simulink model "HM_to_Unity_2013a"  (R2013a)
settings: Solver=FixedStepDiscrete  StartTime=0.0  StopTime=Inf  FixedStep=0.0004  RelTol=1e-3
InitFcn:
  | SampleTime = 0.0004;
  | sampleTime = 0.0004;
undefined symbols (not defined in the file or in its folder): DiscIntNeverNeededParam
libraries: simulink x26, dspsigops x10, xpcmeasurementcomputinglib x7, xpclib x6, dspmtrx3 x4, etargetslib x2, hm_iointerface_lib x2, hm_control_lib x2, sensors_jr3_lib x1
(part 2 of 2)

== matlab function HM_to_Unity_2013a/Subsystem/GotoBlock/compare ==
  data: sig input; f output; comp input; eps input
function f = fcn(sig,comp,eps)
% This block supports the Embedded MATLAB subset.
% See the help menu for details. 

dVec=comp-sig;
delta=norm(dVec);
if (delta<eps)
    f=1;
else
    f=0;
end

== stateflow chart HM_to_Unity_2013a/Robot State Control/Chart2 ==
  state MotorOn1
    en:State=-2;
    en:inPosReset=0;
    count=0;
    du:State=-2;
    du:inPosReset=1;
    ex:inPosReset=0;
  state MotorOn
    en:State=-2;
    count=0;
    du:count=count+1;
    du:State=-2;
  state WaitNewState
    count=0;
    du:count=count+1;
  state DeadMan
    en:State=-1;
    count=0;
    du:State=-1;
  state KeepPos
    en:State=0;
    count=0;
    du:State=0;
    du:count=count+1;
  state FreeSpace
    en:State=1;
    count=0;
    du:State=1;
    du:count=count+1;
  state GoTo1
    en:State=3;
    count=0;
    du:State=3;
    du:count=count+1;
  state Main
    en:State=2;
    count=0;
    du:State=2;
    du:count=count+1;
  state GoTo
    en:State=3;
    count=0;
    du:State=3;
    du:count=count+1;
  (default) -> MotorOn1
  DeadMan -> MotorOn : [DMSwitch==1]
  MotorOn1 -> DeadMan [order 1] : [DMSwitch==0]
  MotorOn -> KeepPos [order 2] : [F0==1 && reset==1]
  MotorOn -> DeadMan [order 1] : [DMSwitch==0]
  MotorOn1 -> KeepPos [order 2] : [F0==1 && reset==1]
  WaitNewState -> KeepPos [order 1] : [F0==1 && reset==1]
  KeepPos -> DeadMan [order 1] : [DMSwitch==0]
  GoTo -> KeepPos [order 1] : [F0==1 && reset==1]
  KeepPos -> WaitNewState [order 2] : [count>2000]
  Main -> KeepPos [order 1] : [F0==1 && reset==1]
  WaitNewState -> FreeSpace [order 2] : [F1==1 && reset==1]
  FreeSpace -> DeadMan [order 1] : [DMSwitch==0]
  FreeSpace -> WaitNewState [order 2] : [count>2000]
  GoTo1 -> DeadMan [order 1] : [DMSwitch==0]
  WaitNewState -> GoTo1 [order 3] : [F2==1 && reset==1]
  GoTo1 -> Main [order 2] : [finishedTask==1]
  GoTo1 -> Main [order 3] : [F2==1 && reset==1 && (count>13000) ]
  Main -> DeadMan [order 2] : [DMSwitch==0]
  WaitNewState -> GoTo [order 4] : [F3==1 && reset==1]
  GoTo -> DeadMan [order 2] : [DMSwitch==0]
  WaitNewState -> DeadMan [order 5] : [DMSwitch==0]
  data: State output double; count local uint32; finishedTask input boolean; F0 input double; F1 input double; F2 input double; F3 input double; reset input double; DMSwitch input double; inPosReset output double =0

== stateflow chart HM_to_Unity_2013a/Robot State Control/Chart1 ==
  state Up
    en:handleType=0
  state Down
    en:handleType=1
  (default) -> Up
  Up -> Down : [Switch==1 && after(1,sec)]
  Down -> Up : [Switch==1 && after(1,sec)]
  data: Switch input; handleType output double

== matlab function HM_to_Unity_2013a/HapticMaster inputs/Balanca enkoderji/Sile na rockah ==
  data: Fd input; Fdo output
function Fdo    = fcn(Fd)
%#codegen

Fdo = Fd;

Fdo(1) = Fd(3);
Fdo(2) = Fd(1);
Fdo(3) = -Fd(2);

% Flo(1) = Fl(2);
% Flo(2) = -Fl(3);
% Flo(3) = Fl(1);
% 
% Fdo(1) = -Fd(2);
% Fdo(2) = Fd(3);
% Fdo(3) = Fd(1);

== matlab function HM_to_Unity_2013a/HapticMaster inputs/Sila_na_vhu/Sila na vrhu ==
  data: rot_mali input; rot_velik input; F output; Fd input
function F   = fcn(rot_mali, rot_velik, Fd)
%#codegen

Rm=[1 0 0;0 cos(rot_velik) -sin(rot_velik);0 sin(rot_velik) cos(rot_velik)];
F=Rm*Fd;

== matlab function HM_to_Unity_2013a/Main ==
  data: Unity_World_Pos output; Unity_Scale output; UnityAngles output; inputWorldPos input; inputMotors input; getJointPos input; TargetNumber input; TargetPos output; Color output; OutputTarget output; State output; ListOfTargets input; ListOfTargetsForSecondExp input; ListOfTarget3rdExp input; NumOfTarRep input; angleofJoint output
function [Unity_World_Pos,Unity_Scale,UnityAngles,TargetPos,Color,OutputTarget,State,angleofJoint]= Main(inputWorldPos,inputMotors,getJointPos,TargetNumber,ListOfTargets,ListOfTargetsForSecondExp,ListOfTarget3rdExp,NumOfTarRep)
% This block supports the Embedded MATLAB subset.
% See the help menu for details. 
 State = -1;

Color=0;

%Converting axis
aim_x = inputWorldPos(2);
aim_y = inputWorldPos(3);
scaleofAim = inputWorldPos(1);

%Deviation of angles from handle
anglefor2nd = inputMotors(1);
angleofAim = inputMotors(2);

joint_y = getJointPos(2);
joint_x = getJointPos(1);
if (joint_y < 0)
    joint_y=joint_y;
end


%angleofJoint =atan (joint_y/joint_x)*180/pi;

angleofJoint = joint_y*180/pi;


Unity_X= aim_x ;
Unity_Y = aim_y ;
%Unity_Scale  = (scaleofAim*100)+23;
Unity_Scale= scaleofAim;
angleofAim = angleofAim* 180/pi;
anglefor2nd = anglefor2nd *180/pi;



Unity_World_Pos =[Unity_X,Unity_Y];



%Third row means angle of object and 4th one means scale of object
%%ListOfTargets=[FirstT_x,FirstT_y,30,1;SecondT_x,SecondT_y,0,1.5;ThirdT_x,ThirdT_y,0,1;FourT_x,FourT_y,0,1];
%ListOfTargets=[4.1,-3.7;5.5,-4];
%ExpType=ExpT;

% ka =1;
% if (ka ==1)
% NumberOfTarget = NumOfTarRep (1);
% NumberOfRepeatation = NumOfTarRep (2);
% %size=NumberOfTarget*5;
% OutputTarget = zeros (NumberOfTarget,NumberOfRepeatation);
% else
%     OutputTarget = zeros (1,1);
% end

Deviation = NumOfTarRep(4);
DeviationForScale = NumOfTarRep(5);
DevForAngle=NumOfTarRep(6);
DevForAngle2=NumOfTarRep(7);

ExpType =NumOfTarRep (3);

if (ExpType==1)
    
    UnityAngles = [angleofAim,anglefor2nd];
    OutputTarget = ListOfTargets;
    TargetPos = ListOfTargets (TargetNumber,:);
    if ((Unity_X >TargetPos(1)-Deviation) && ( Unity_Y>TargetPos(2)-Deviation) && (Unity_X<TargetPos(1)+Deviation) && (Unity_Y<TargetPos(2)+Deviation) && (Unity_Scale<TargetPos(4)+DeviationForScale) && (Unity_Scale > TargetPos(4)-DeviationForScale)&&(angleofAim <TargetPos(3)+DevForAngle)&&(angleofAim >TargetPos(3)-DevForAngle))
    %|| (colorCounter>=1 && 100>colorCounter)

State = 1;
Color=1;
%colorCounter = colorCounter+1;
%else
 %   colorCounter =0;
    
elseif (Unity_Scale<TargetPos(4)+DeviationForScale) && (Unity_Scale > TargetPos(4)-DeviationForScale)
    
    Color=2;
   end
elseif (ExpType==3)
    
    limit = anglefor2nd+angleofJoint;
    if (limit > 28)
        limit =28;
    else if (limit < -28)
            limit = -28;
        end
    end
    UnityAngles = [angleofAim,limit];
    OutputTarget = ListOfTarget3rdExp;
    TargetPos = ListOfTarget3rdExp(TargetNumber,:);
    if ((Unity_X >TargetPos(1)-Deviation) && ( Unity_Y>TargetPos(2)-Deviation) && (Unity_X<TargetPos(1)+Deviation) && (Unity_Y<TargetPos(2)+Deviation) && (Unity_Scale<TargetPos(4)+DeviationForScale) && (Unity_Scale > TargetPos(4)-DeviationForScale)&&(angleofAim <TargetPos(3)+DevForAngle)&&(angleofAim >TargetPos(3)-DevForAngle)&&(limit <TargetPos(5)+DevForAngle2)&&(limit >TargetPos(5)-DevForAngle2)) 
    %|| (colorCounter>=1 && 100>colorCounter)

State = 1;
Color=1;
    
elseif (Unity_Scale<TargetPos(4)+DeviationForScale) && (Unity_Scale > TargetPos(4)-DeviationForScale)
    
    Color=2;
   end
elseif (ExpType==2)
    
    limit2=anglefor2nd+(angleofJoint);
    if (limit2 > 26)
        limit2=26;
    else if (limit2 < -26)
            limit2 = -26;
        end
    end
    UnityAngles = [angleofAim,limit2];
    OutputTarget = ListOfTargets;
    TargetPos = ListOfTargetsForSecondExp(TargetNumber,:);
    if ((Unity_X >TargetPos(1)-Deviation) && ( Unity_Y>TargetPos(2)-Deviation) && (Unity_X<TargetPos(1)+Deviation) && (Unity_Y<TargetPos(2)+Deviation) && (Unity_Scale<TargetPos(4)+DeviationForScale) && (Unity_Scale > TargetPos(4)-DeviationForScale)&&(angleofAim <TargetPos(3)+DevForAngle)&&(angleofAim >TargetPos(3)-DevForAngle)&&(limit2 <TargetPos(5)+DevForAngle2)&&(limit2 >TargetPos(5)-DevForAngle2)) 
    %|| (colorCounter>=1 && 100>colorCounter)

State = 1;
Color=1;
    
elseif (Unity_Scale<TargetPos(4)+DeviationForScale) && (Unity_Scale > TargetPos(4)-DeviationForScale)
    
    Color=2;
   end
else
    
    UnityAngles = [angleofAim,anglefor2nd];
    OutputTarget = ListOfTargets;
    TargetPos = ListOfTargets (TargetNumber,:);
end


%NumberOfTarget = NumOfTarRep (1);
%NumberOfRepeatation = NumOfTarRep (2);
%size=NumberOfTarget*5;
%PosOfTargets = zeros (1,1);
%PosOfTargets = zeros (size,1);
%k=1;
%for x =1:NumberOfTarget
 %   for c = 1:5
 
%PosOfTargets(k,1) = ListOfTargets(x,c);
%k=k+1;
 %   end
%end

%colorCounter =1;

== stateflow chart HM_to_Unity_2013a/Chart ==
  state State01
    en:TargetNumber=1;
    du:TargetNumber=1;
    en:repeat =0;
    Triger=0;
    Triger2=0;
  state State0
    en:TargetNumber=1;
    du:TargetNumber=1;
    en:repeat =0;
    Triger=0;
    Triger2=0;
  state Finish1
    TargetNumber=-1;
  state WaitNewState2
    count=0;
    du:count=count+1;
    Triger=1;
    Triger2=1;
  state Not
    Triger=0;
  state State
    TargetNumber =TargetNumber+1;
    Triger2=0;
  state x1
    repeat=repeat+1;
    TargetNumber=0;
  state WaitNewState3
    count=0;
    du:count=count+1;
  state WaitNewState
    count=0;
    du:count=count+1;
  state Finish
    TargetNumber=-1;
  state WaitNewState1
    count=0;
    du:count=count+1;
  state State1
    TargetNumber =TargetNumber+1;
  state x
    repeat=repeat+1;
    TargetNumber=1
  state State2
    TargetNumber =TargetNumber+1;
  state State3
  (default) -> State01
  State01 -> State0 : [MainState==1]
  Finish1 -> State0 : [Reset==1 || ExpType ==1]
  State -> State0 [order 2] : [Reset==1 || ExpType ==1]
  State0 -> WaitNewState2 : [State==1  ]
  x1 -> Finish1 [order 1] : [repeat==NumberOfRepetation]
  State -> WaitNewState2 [order 3] : [State==1]
  WaitNewState2 -> Not : [count ==6750]
  Not -> WaitNewState3 : [State==1]
  x1 -> State [order 2] : [repeat!=NumberOfRepetation]
  State -> x1 [order 1] : [TargetNumber==NumOfTarget+1 ]
  WaitNewState3 -> State : [count ==750]
  x -> Finish [order 2] : [repeat==NumberOfRepetation]
  WaitNewState1 -> State1 : [count==7500]
  State1 -> WaitNewState [order 1] : [State==1]
  State1 -> x [order 2] : [TargetNumber==NumOfTarget+1 ]
  x -> WaitNewState1 [order 1] : [State==1]
  WaitNewState -> State1 [order 1] : [count==7500]
  State2 -> x [order 2] : [TargetNumber==NumOfTarget +1]
  WaitNewState -> State2 [order 2] : [count==7500]
  State2 -> WaitNewState [order 1] : [State==1]
  data: TargetNumber output double; State input double; count local double; NumOfTarget input double; NumberOfRepetation input; Triger output double; Triger2 output double; repeat output double; Reset input double; ExpType input double; MainState input double

== matlab function HM_to_Unity_2013a/Subsystem/Main/Task/vector4 ==
  data: u input; y output
function y = trans(u)
% This block supports the Embedded MATLAB subset.
% See the help menu for details. 

y =[u(1);u(2);u(3)];

== stateflow chart HM_to_Unity_2013a/ExpType ==
  state State0
    en:expType =1;
    du:expType=1;
  state State12
    count =0;
    du:count=count+1;
  state State23
    count =0;
    du:count=count+1;
  state State22
    count =0;
    du:count=count+1;
  state State11
    expType=2;
    du:count=count+1;
  state State21
    expType=3;
    en:count=0;
    du:count=count+1;
  (default) -> State0
  State23 -> State0 : [count ==2500]
  State0 -> State12 : [State==1]
  State12 -> State11 : [count ==2500]
  State21 -> State23 : [State==1]
  State11 -> State22 : [State==1]
  State22 -> State21 : [count ==2500]
  data: expType output double; State input double; count local double

== matlab function HM_to_Unity_2013a/trgSum  ==
  data: trg input; y output; trg2 input; trg3 input; trg4 input
function y = trans(trg,trg2,trg3,trg4)

% This block supports the Embedded MATLAB subset.
% See the help menu for details. 

y =[trg,trg2,trg3,trg4];

== matlab function HM_to_Unity_2013a/Subsystem/GotoBlock/runGoTo/Embedded MATLAB Function ==
  data: p0 input; p output; v0 input; pk input; vk input; T input; t input; v output
function [p,v] = f_runGoTo(p0,v0,pk,vk,T,t)
%vhod 	p0,v0,pk,vk,T,t
%izhod p,v

%p0=10;,v0=2;,pk=0;,vk=0;,T=3;,t=0:0.01:T;

a0=p0;
a1=v0;
a2=(3/(T*T))*(pk-p0)-(2/T)*v0-(1/T)*vk;
a3=(-2/(T*T*T))*(pk-p0)+(1/(T*T))*(vk+v0);

%p=a3*t.*t.*t+a2*t.*t+a1*t+a0;
%v=3*a3*t.*t+2*a2*t+a1;
p=a3*t*t*t+a2*t*t+a1*t+a0;
v=3*a3*t*t+2*a2*t+a1;

if (t>T)
    p=pk;
    v=vk;
end

== matlab function HM_to_Unity_2013a/Subsystem/Main/Task/vector1 ==
  data: u input; y output
function y = trans(u)
% This block supports the Embedded MATLAB subset.
% See the help menu for details. 

y =[u(1);u(2);u(3)];

== matlab function HM_to_Unity_2013a/HapticMaster inputs/vector4 ==
  data: u input; y output
function y = trans(u)
% This block supports the Embedded MATLAB subset.
% See the help menu for details. 

y =[u(1),u(2),u(3)];

== matlab function HM_to_Unity_2013a/HapticMaster inputs/vector5 ==
  data: u input; y output
function y = trans(u)
% This block supports the Embedded MATLAB subset.
% See the help menu for details. 

y =[u(1),u(2),u(3)];

== matlab function HM_to_Unity_2013a/HapticMaster outputs/LED ==
  data: L1 output; L2 output; L3 output; state input; handleType input; L4 output; L5 output; L6 output; L7 output; L8 output; time input
function [L1,L2,L3,L4,L5,L6,L7,L8] = LED(state,handleType,time)
% This block supports the Embedded MATLAB subset.
% See the help menu for details. 

L1=0;
L2=0;
L3=0;
L4=0;
L5=0;
L6=0;
L7=0;
L8=0;

switch (state)
    case(-2)
        if (mod(round(time),2)==1)
        L5=1;
        L6=1;
        L7=1;
        L8=1;
        end
    case(-1)
        if (mod(round(time),2)==1)
        L1=1;
        L2=1;
        L3=1;
        L4=1;
        end
    case(0)
        L6=1;
    case(1)
        L2=1;
        L7=1;
    case(2)
        L6=1;
    case(3)
        L5=1;
    case(4)
        L2=1;
end

if (handleType)
    L8=1;
end

== stateflow chart HM_to_Unity_2013a/Subsystem/KeepPosBlock/Chart ==
  state Inactive
    en:InternalState=-1;
  state Init
    en:InternalState=0;
    finished=0;
  state Running
    du:InternalState=1;
  state positionReached
    en:InternalState=2;
    finished=1;
  (default) -> Inactive
  Inactive -> Init : [State==0]
  Init -> Running : [InternalState==0]
  Running -> positionReached : [posReached==1]
  data: State input; InternalState output double; posReached input; finished output boolean

== matlab function HM_to_Unity_2013a/Subsystem/Main/Task/vector2 ==
  data: u input; y output
function y = trans(u)
% This block supports the Embedded MATLAB subset.
% See the help menu for details. 

y =[u(1);u(2);u(3)];

== matlab function HM_to_Unity_2013a/HapticMaster inputs/InitPosition ==
  data: u input; y output
function y = inPos(u)
% This block supports the Embedded MATLAB subset.
% See the help menu for details. 

y=[0; 0; 0];

%1.joint
x11=4.11;
x12=-7.70;

y11=-0.19;% metri
y12=0.19;% metri

k1=(y11-y12)/(x11-x12);
d1=y12-k1*x12;

y(1) = k1 * u(1) + d1;

%2.joint
x21=-4.24;
x22=-2.55;

y21=-0.504;% radiani
y22=0.507;% radiani

k2=(y21-y22)/(x21-x22);
d2=y22-k2*x22;

y(2) = k2 * u(2) + d2;

%3.joint
x31=-7.86;
x32=6.16;

y31=-0.228;% metri
y32=0.228;% metri

k3=(y31-y32)/(x31-x32);
d3=y32-k3*x32;

y(3) = k3 * u(3) + d3; 
%y(3) = -0.228;
